simulink model "Rate_Transition"  (R2025b)
settings: Solver=FixedStepDiscrete  StartTime=0.0  StopTime=10.0  FixedStep=0.005  RelTol=1e-3
settings Model: Creator=soura  LastModifiedBy=soura
settings DebuggingCC: TimeAdjustmentMsg=warning  InheritedTsInSrcMsg=error

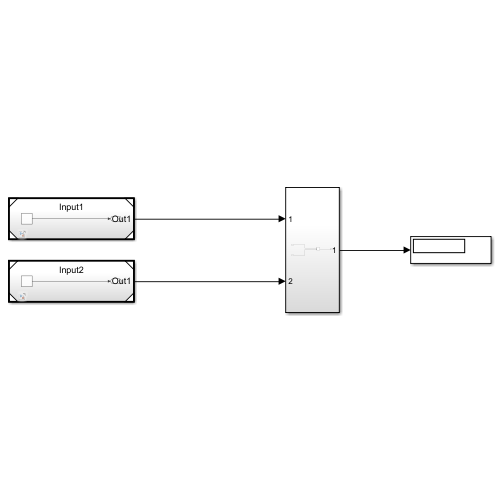
[thumbnail: Simulink's stored preview of the top-level diagram]
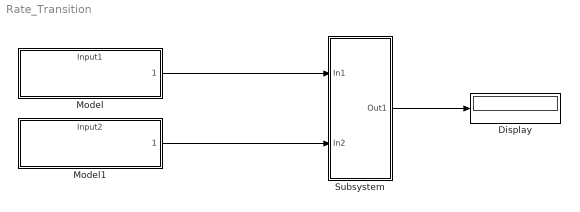
== system Rate_Transition ==
  Display : Display
  Model : ModelReference  ModelNameDialog=Input1.slx  SimulationMode=Normal  ModelReferenceVersion=1.7  InputSignalHandling=Zero-order hold  OutputSignalHandling=Zero-order hold
  Model1 : ModelReference  ModelNameDialog=Input2.slx  SimulationMode=Normal  ModelReferenceVersion=1.6
  Subsystem : Subsystem
  wires:
  Subsystem/1(Out1) -> Display/1
  Model/1 -> Subsystem/1(In1)
  Model1/1 -> Subsystem/2(In2)

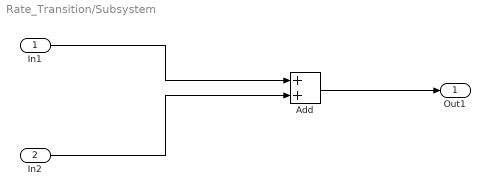
== system Rate_Transition/Subsystem ==
  In1 : Inport
  In2 : Inport  Port=2
  Add : Sum
  Out1 : Outport
  wires:
  In2/1 -> Add/2
  Add/1 -> Out1/1
  In1/1 -> Add/1
